simulink model "simularePIcontinuu"  (R2022b)
settings: Solver=VariableStepAuto  StartTime=0.0  StopTime=30  RelTol=1e-3
settings Model: Creator=saioc  LastModifiedBy=saioc
settings ModelReferenceCC: EnableRefExpFcnMdlSchedulingChecks=on

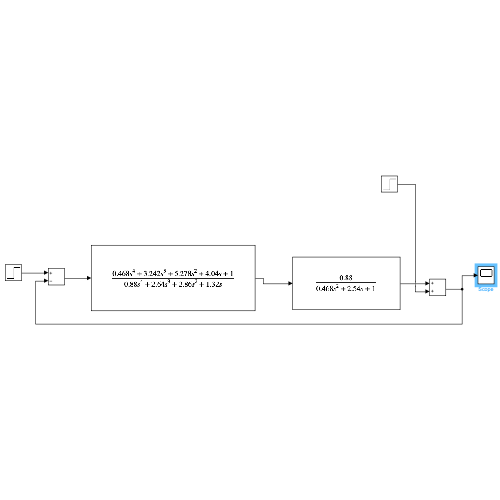
[thumbnail: Simulink's stored preview of the top-level diagram]
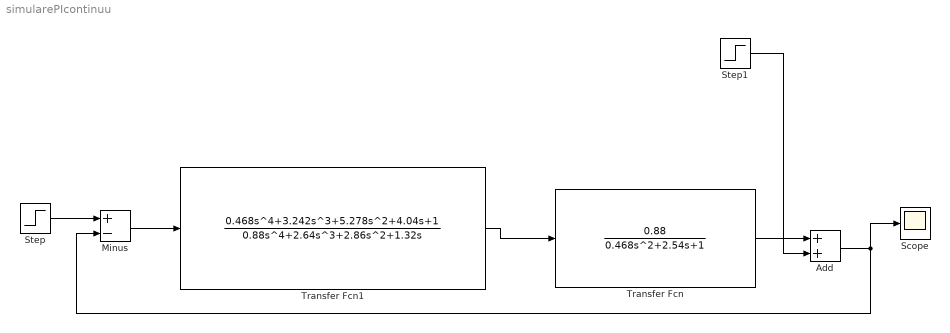
== system simularePIcontinuu ==
  Add : Sum
  Minus : Sum  Inputs=+-
  Scope : Scope
  Step : Step  Time=0  After=150
  Step1 : Step  Time=15  After=100
  Transfer Fcn : TransferFcn  Numerator=[0.88]  Denominator=[0.468 2.54 1]
  Transfer Fcn1 : TransferFcn  Numerator=[0.468 3.242 5.278 4.04 1]  Denominator=[0.88 2.64 2.86 1.32 0]
  wires:
  Step/1 -> Minus/1
  Minus/1 -> Transfer Fcn1/1
  Transfer Fcn1/1 -> Transfer Fcn/1
  Step1/1 -> Add/2
  Transfer Fcn/1 -> Add/1
  Add/1 -> Minus/2, Scope/1
